simulink model "DoubleInvertedPendulum_StateFeedback"  (R2015a)
settings: Solver=ode45  StartTime=0.0  StopTime=20  RelTol=1e-3
values from neighbouring files (symbols this model uses):
  gain = lqr( A ,B, Q, R )    [DoubleInvertedPendulum_config.m]
settings Model: Creator=hamada  LastModifiedBy=hamada

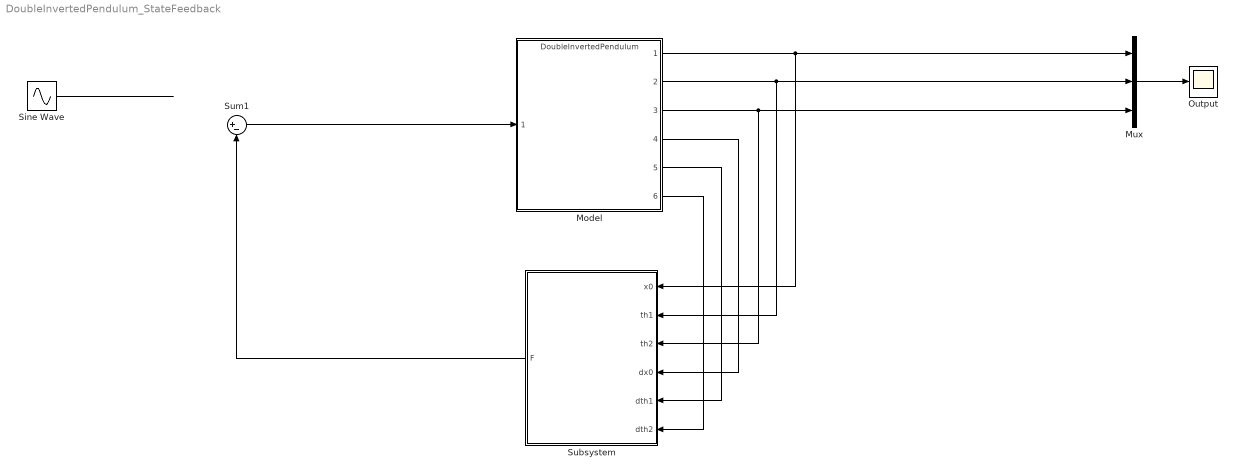
== system DoubleInvertedPendulum_StateFeedback ==
  Model : ModelReference  ModelNameDialog=DoubleInvertedPendulum  SimulationMode=Normal  ModelReferenceVersion=1.2  CopyOfModelName=DoubleInvertedPendulum  DefaultDataLogging=on
  Mux : Mux  Inputs=3
  Output : Scope
      settings: SaveName=Output  SampleInput=on  SampleTime=dSamplingPeriod
  Sine Wave : Sin  Amplitude=10  Frequency=1*2*pi  SampleTime=0
  Subsystem : Subsystem
  Sum1 : Sum  Inputs=|+-
  wires:
  Sine Wave/1 -> ?
  Mux/1 -> Output/1
  Subsystem/1(F) -> Sum1/2
  Sum1/1 -> Model/1
  Model/1 -> Mux/1, Subsystem/1(x0)
  Model/2 -> Mux/2, Subsystem/2(th1)
  Model/3 -> Mux/3, Subsystem/3(th2)
  Model/4 -> Subsystem/4(dx0)
  Model/5 -> Subsystem/5(dth1)
  Model/6 -> Subsystem/6(dth2)

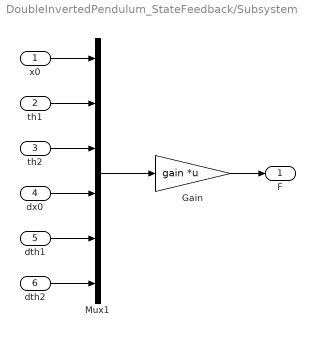
== system DoubleInvertedPendulum_StateFeedback/Subsystem ==
  x0 : Inport
  th1 : Inport  Port=2
  th2 : Inport  Port=3
  dx0 : Inport  Port=4
  dth1 : Inport  Port=5
  dth2 : Inport  Port=6
  Gain : Gain  Gain=gain  Multiplication=Matrix(K*u)
  Mux1 : Mux  Inputs=6
  F : Outport
  wires:
  Mux1/1 -> Gain/1
  dth2/1 -> Mux1/6
  dx0/1 -> Mux1/4
  th1/1 -> Mux1/2
  dth1/1 -> Mux1/5
  x0/1 -> Mux1/1
  th2/1 -> Mux1/3
  Gain/1 -> F/1
